simulink model "model5"  (R2024b)
settings: Solver=VariableStepAuto  StartTime=0.0  StopTime=10.0  RelTol=1e-3
undefined symbols (not defined in the file): B, g, N, x0, y0, z0
settings Model: Creator=kacpe  LastModifiedBy=kacpe

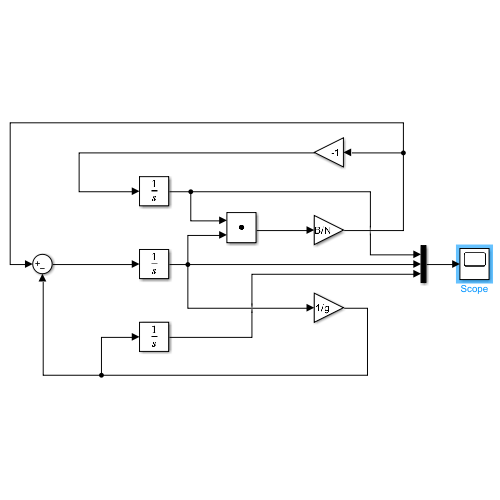
[thumbnail: Simulink's stored preview of the top-level diagram]
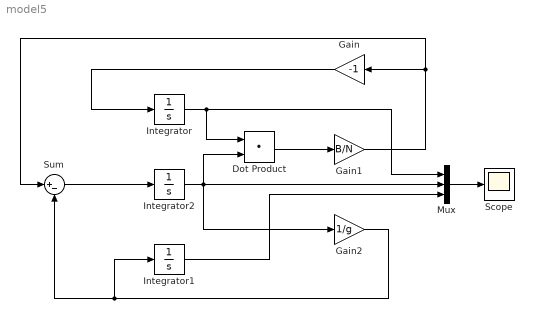
== system model5 ==
  Dot Product : DotProduct  OutDataTypeStr=Inherit: Inherit via internal rule
  Gain : Gain  Gain=-1
  Gain1 : Gain  Gain=B/N
  Gain2 : Gain  Gain=1/g
  Integrator : Integrator  InitialCondition=x0
  Integrator1 : Integrator  InitialCondition=z0
  Integrator2 : Integrator  InitialCondition=y0
  Mux : Mux  Inputs=3
  Scope : Scope
  Sum : Sum  Inputs=|+-
  wires:
  Gain/1 -> Integrator/1
  Integrator/1 -> Mux/1, Dot Product/1
  Integrator2/1 -> Mux/2, Dot Product/2, Gain2/1
  Gain1/1 -> Sum/1, Gain/1
  Gain2/1 -> Integrator1/1, Sum/2
  Integrator1/1 -> Mux/3
  Sum/1 -> Integrator2/1
  Dot Product/1 -> Gain1/1
  Mux/1 -> Scope/1
